simulink model "driver_model_b_upd (2)"  (R2023a)
settings: Solver=FixedStepDiscrete  StartTime=0  StopTime=700  FixedStep=0.0005  RelTol=1e-3  AbsTol=1e-6
InitFcn:
  | R2D = 180/pi;
undefined symbols (not defined in the file or in its folder): b_hat_Max, SrsLrn_BrkPedDownLim, SrsLrn_BrkPedUpLim, SrsLrn_EKF_Q1, SrsLrn_EKF_Q2, SrsLrn_ExitAccPedLim, SrsLrn_Lamda1, SrsLrn_Lamda2, SrsLrn_LongAccDownLim, SrsLrn_LongAccUpLim, SrsLrn_State1Cnt, SrsLrn_State2Cnt, SrsLrn_State5Cnt, SrsLrn_State6Cnt, SrsLrn_State7Cnt, SrsLrn_UpdBrkPedDown, SrsLrn_UpdBrkPedUp, tau_hat_Max
libraries: simulink x11, slpidlib x2, Solver_SF x1
(part 2 of 2)

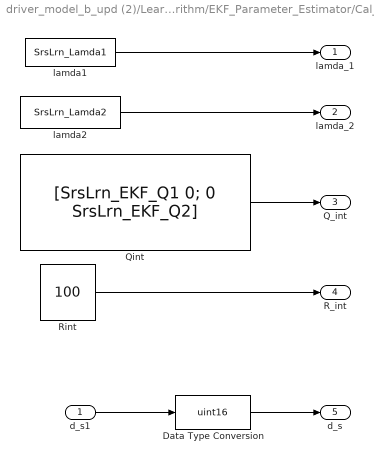
== system driver_model_b_upd (2)/LearningAlgorithm/EKF_Parameter_Estimator/Cal_para ==
  d_s1 : Inport
  Data Type Conversion : DataTypeConversion  OutDataTypeStr=uint16  SaturateOnIntegerOverflow=off  RndMeth=Floor
  Qint : Constant  Value=[SrsLrn_EKF_Q1 0; 0 SrsLrn_EKF_Q2]  OutDataTypeStr=fixdt(0,16,0.001,0)
  Rint : Constant  Value=100  OutDataTypeStr=fixdt(0,16,2)
  lamda1 : Constant  Value=SrsLrn_Lamda1
  lamda2 : Constant  Value=SrsLrn_Lamda2
  lamda_1 : Outport
  lamda_2 : Outport  Port=2
  Q_int : Outport  Port=3
  R_int : Outport  Port=4
  d_s : Outport  Port=5
  wires:
  lamda1/1 -> lamda_1/1
  Rint/1 -> R_int/1
  Qint/1 -> Q_int/1
  lamda2/1 -> lamda_2/1
  d_s1/1 -> Data Type Conversion/1
  Data Type Conversion/1 -> d_s/1

== stateflow chart driver_model_b_upd (2)/LearningAlgorithm/EKF_Parameter_Estimator/Initialize ==
  state Initialize
    en: y=0;
  state AfterInit
    en: y=1;
  (default) -> Initialize
  Initialize -> AfterInit
  data: y output

== stateflow chart driver_model_b_upd (2)/Chart ==
  state Accel_INIT_ON
    en:
    driver = uint8(0);
    srs =uint8(0);
    accel =uint8(0);
    accel_init = uint8(1);
  state SRS_ON
    en:
    driver = uint8(0);
    srs = uint8(1);
    SRSCnt=uint16(1);
    du:
    SRSCnt=SRSCnt+1;
    ex:
    SRSCnt=uint16(0);
  state Driver_ON
    en:
    driver = uint8(1);
    srs = uint8(0);
    DriverCnt=uint16(1);
    du:
    DriverCnt=DriverCnt+1;
    ex:
    DriverCnt=uint16(0);
  state Loop_State
    en:
    Loop=uint16(1);
    PreLoop = uint16(1);
  state INIT
    en:
    driver = uint8(0);
    srs =uint8(0);
    accel = uint8(0);
    accel_init = uint8(0);
    SRSCheck = uint16(0);
    DriverCnt=uint16(0);
  state Accel_ON
    en:
    driver = uint8(0);
    srs =uint8(0);
    accel = uint8(1);
    ACCCnt=uint16(1);
    du:
    ACCCnt=ACCCnt+1;
    ex:
    ACCCnt=uint16(0);
  state Loop_Update
    en:
    PreLoop = Loop;
    Loop=Loop+1;
    LoopCnt=uint16(1);
    du:
    LoopCnt=LoopCnt+1;
    ex:
    LoopCnt=uint16(0);
  state OFF
    en:
    driver = uint8(0);
    srs =uint8(0);
    accel = uint8(0);
  state Accel_OFF
    en:
    driver = uint8(0);
    srs =uint8(0);
    accel = uint8(0);
    ACCCnt=uint16(1);
    du:
    ACCCnt=ACCCnt+1;
    ex:
    ACCCnt=uint16(0);
  state Accel_INIT_OFF_L
    en:
    driver = uint8(0);
    srs =uint8(0);
    accel = uint8(0);
  state SRS_ON_L
    en:
    driver = uint8(0);
    srs = uint8(1);
    accel = uint8(0);
    SRSCnt=uint16(1);
    du:
    SRSCnt=SRSCnt+1;
    ex:
    SRSCnt=uint16(0);
  state Driver_ON_L
    en:
    driver = uint8(1);
    srs = uint8(0);
    accel = uint8(0);
    DriverCnt=uint16(1);
    du:
    DriverCnt=DriverCnt+1;
    ex:
    DriverCnt=uint16(0);
  state Accel_INIT_L
    en:
    driver = uint8(0);
    srs =uint8(0);
    accel = uint8(1);
    ACCCnt=uint16(1);
    du:
    ACCCnt=ACCCnt+1;
    ex:
    ACCCnt=uint16(0);
  state Accel_ON_L
    en:
    driver = uint8(0);
    srs =uint8(0);
    accel = uint8(1);
    ACCCnt=uint16(1);
    du:
    ACCCnt=ACCCnt+1;
    ex:
    ACCCnt=uint16(0);
  state Loop_Update_L
    en:
    PreLoop = Loop;
    Loop=Loop+1;
  state OFF_Driver_L
    en:
    driver = uint8(0);
    srs =uint8(0);
    accel = uint8(0);
  state Accel_OFF_L
    en:
    driver = uint8(0);
    srs =uint8(0);
    accel = uint8(0);
  (default) -> Loop_State
  SRS_ON -> Driver_ON : [(v_ego <1 && SRSCnt > 200) ||...
      |  (Pre_Vehicle_speed - v_ego >= 0 &&...
      |  SRSCnt > 200 ) ||...
      |  (d_des_driver > delta_d &&...
      |  SRSCnt > 200 )]
  INIT -> Accel_INIT_ON [order 2] : [Loop == 1 &&...
      |  D_des_SRS < delta_d &&...
      |  clock >=0]
  Accel_INIT_ON -> SRS_ON : [throttle_input == 0 &&...
      | Pre_Vehicle_speed - v_ego < 0  &&...
      |  D_des_SRS > delta_d ]
  Loop_State -> INIT
  Driver_ON -> OFF : [(d_des_driver <= delta_d  &&...
      |  clock < 100 &&...
      | DriverCnt > 50) ||...
      | clock >= 100*Loop]
  OFF -> Driver_ON [order 1] : [Pre_Vehicle_speed - v_ego < 3 &&...
      | d_des_driver > delta_d  &&...
      | clock <100 *Loop  ]
  Accel_ON -> INIT [order 2] : [clock >= 200*PreLoop]
  OFF -> Loop_Update [order 2] : [clock >=100*Loop]
  Accel_ON -> Accel_OFF [order 1] : [( v_ego - Pre_Vehicle_speed  > 3 &&...
      |  ACCCnt >100 ) ||...
      |  delta_d <= 15  ]
  Accel_OFF -> Accel_ON [order 1] : [D_des_SRS < delta_d &&...
      | clock >= 100 &&...
      | delta_d >=70]
  Loop_Update -> (junction 292)
  (junction 292) -> Accel_OFF
  Accel_OFF -> INIT [order 2] : [clock >= PreLoop*200]
  Accel_INIT_OFF_L -> (junction 288) [order 1] : [Pre_Vehicle_speed - v_ego < 0  &&...
      |  D_des_SRS > delta_d]
  (junction 288) -> SRS_ON_L
  Accel_INIT_OFF_L -> Accel_INIT_L [order 2] : [D_des_SRS < delta_d &&...
      | delta_d > 80]
  Accel_INIT_L -> Accel_INIT_OFF_L : [ACCCnt == 200 ||...
      |  delta_d < 10 ||...
      | D_des_SRS +20 >= delta_d ||...
      | (v_ego >=18 && ACCCnt == 200)]
  SRS_ON_L -> Driver_ON_L : [(v_ego <1 && SRSCnt >100) ||...
      |  (Pre_Vehicle_speed - v_ego <= 0 &&...
      | d_des_driver >= delta_d &&...
      |  SRSCnt > 100) ||...
      |  (d_des_driver > delta_d &&...
      |  SRSCnt > 100 )]
  INIT -> Accel_INIT_L [order 1] : [Loop == (PreLoop+1)&&...
      |  D_des_SRS <= delta_d &&...
      | clock >=100*Loop]
  (junction 211) -> SRS_ON_L
  Driver_ON_L -> OFF_Driver_L : [(d_des_driver <= delta_d &&...
      | DriverCnt > 50 &&...
      | Pre_Vehicle_speed - v_ego >= 0 &&...
      | clock < (100+PreLoop*200))||...
      | clock >= (100+PreLoop*200) ||...
      | d_des_driver <= delta_d ]
  OFF_Driver_L -> Driver_ON_L [order 2] : [(clock < (100+PreLoop*200) &&...
      |  Pre_Vehicle_speed - v_ego < 0 &&...
      |  d_des_driver > delta_d )]
  INIT -> (junction 211) [order 3] : [Loop==(PreLoop+1) &&...
      | Pre_Vehicle_speed - v_ego < 0  &&...
      |  D_des_SRS > delta_d &&...
      |  clock >=100*Loop + 15]
  Accel_ON_L -> INIT [order 2] : [clock >=PreLoop*200]
  OFF_Driver_L -> Loop_Update_L [order 1] : [clock >=200*PreLoop+100]
  Accel_ON_L -> Accel_OFF_L [order 1] : [(v_ego - Pre_Vehicle_speed  > 3 &&...
      | clock < PreLoop*200 &&...
      |  ACCCnt >100 ) ||...
      |  (clock < PreLoop*200 &&...
      | delta_d < 15) ]
  Accel_OFF_L -> Accel_ON_L [order 1] : [D_des_SRS < delta_d &&...
      | clock < PreLoop*200 &&...
      | delta_d >=70]
  Loop_Update_L -> (junction 290)
  (junction 290) -> Accel_OFF_L
  Accel_OFF_L -> INIT [order 2] : [clock >=PreLoop*200]
  data: d_des_driver input; srs output; driver output; accel output; v_ego input; D_des_SRS input; delta_d input; Pre_Vehicle_speed input; DriverCnt local; throttle_input input; SRSCnt local; SRSCheck local; clock input; ACCCnt local; accelCheck local; LoopCnt local; accel_init local; BrakeCnt local; Loop output; DoCnt local; STCnt local; PreLoop local

== stateflow chart driver_model_b_upd (2)/LearningAlgorithm/EKF_Parameter_Estimator/Initialize1 ==
  state Initialize
    en: y=0;
  state AfterInit
    en: y=1;
  (default) -> Initialize
  Initialize -> AfterInit
  data: y output

== stateflow chart driver_model_b_upd (2)/LearningAlgorithm/SRS_Learning_State ==
  state SRSBrkLrnEna
    en:
    SrsLrn_state=uint8(5);
  state Init
    en:
    SrsLrn_state=uint8(0);
  state SRSBrk_ConsAcc
    en:
    BCCnt = uint16(1);
    du:
    BCCnt = BCCnt + 1;
    ex:
    BCCnt = uint16(0);
    state BrkTau_Update
      en:
      SrsLrn_state=uint8(3);
    state Brkb_Update
      en:
      SrsLrn_state=uint8(4);
    (default) -> (junction 94)
    (junction 94) -> BrkTau_Update [order 1] : [RelSpdDivVego < 0.01]
    (junction 94) -> Brkb_Update [order 2] : [RelSpdDivVego > 0.01]
  note: % Brake Pedal 변화 3%미만, Acc 변화 50% 미만
      | [DBCnt > SrsLrn_State2Cnt &&...
      | StrkDpthPcVal < SrsLrn_BrkPedUpLim*BrkStrk &&...
      | StrkDpthPcVal > SrsLrn_BrkPedDownLim*BrkStrk]
      |
      | % 종방향 가속도 조건은 필요시 추가 (종방향 가속도 음수 상황)
      | % LongAccFil > SrsLrn_LongAccDownLim*AccVal &&...
      | % LongAccFil < SrsLrn_LongAccUpLim*AccVal]
  state SRSDriverBrk
    en:
    SrsLrn_state=uint8(2);
    DBCnt = uint16(1);
    BrkStrk = StrkDpthPcVal;
    % AccVal = LongAccFil;
    du:
    DBCnt = DBCnt + 1;
    ex:
    DBCnt = uint16(0);
  state SRSCarfollow
    en:
    SrsLrn_state=uint8(1);
    CfCnt = uint16(1);
    du:
    CfCnt = CfCnt + 1;
    ex:
    CfCnt = uint16(0);
  state SRSDriverAcc
    en:
    SrsLrn_state=uint8(6);
    DBCnt_Acc= uint16(1);
    AccVal = LongAccFil;
    du:
    DBCnt_Acc = DBCnt_Acc + 1;
    ex:
    DBCnt_Acc = uint16(0);
  state SRSAcc_AccUp
    en:
    SrsLrn_state=uint8(7);
    BCCnt_Acc = uint16(1);
    du:
    BCCnt_Acc = BCCnt_Acc + 1;
    ex:
    BCCnt_Acc = uint16(0);
  state SRSAccLrnEna
    en:
    AccCnt = uint16(1);
    AccPed = AccPedDepVal;
    du:
    AccCnt = AccCnt + 1;
    ex:
    AccCnt = uint16(0);
    state AccTau_Update
      en:
      SrsLrn_state=uint8(8);
    state Accb_Update
      en:
      SrsLrn_state=uint8(9);
    (default) -> (junction 100)
    (junction 100) -> AccTau_Update [order 1] : [RelSpdDivVego < 0.05]
    (junction 100) -> Accb_Update [order 2] : [RelSpdDivVego > 0.05]
  (default) -> Init
  SRSBrkLrnEna -> Init : [SmartRegenRdrCstActSta ==0 ||...
      |  AccPedDepVal > 2 ||...
      | ObjDstVal > 100 ||...
      | sEstSpdFilt < 0.5 ||...
      | StrkDpthPcVal > 0.5 ||...
      | ObjRelSpdVal > 0.1]
  SRSBrk_ConsAcc -> SRSBrkLrnEna [order 1] : [StrkDpthPcVal == 0]
  SRSBrk_ConsAcc -> Init [order 2] : [SmartRegenRdrCstActSta ==0 ||...
      |  AccPedDepVal > 2 ||...
      | ObjDstVal > 100 ||...
      | sEstSpdFilt < 0.5 ||...
      | ObjRelSpdVal > 0.1 ||...
      | StrkDpthPcVal > 1.5*BrkStrk ||...
      | StrkDpthPcVal < 0.5*BrkStrk]
      | % 종방향 가속도 조건은 필요시 추가 (종방향 가속도 음수 상황)
      | % LongAccFil < SrsLrn_LongAccDownLim*AccVal ||...
      | % LongAccFil > SrsLrn_LongAccUpLim*AccVal
  SRSDriverBrk -> SRSBrk_ConsAcc [order 2] : % Brake Pedal 변화 3%미만, Acc 변화 50% 미만
      | [DBCnt > SrsLrn_State2Cnt &&...
      | StrkDpthPcVal < 1.5*BrkStrk &&...
      | StrkDpthPcVal > 0.2*BrkStrk]
      |
      | % 종방향 가속도 조건은 필요시 추가 (종방향 가속도 음수 상황)
      | % LongAccFil > SrsLrn_LongAccDownLim*AccVal &&...
      | % LongAccFil < SrsLrn_LongAccUpLim*AccVal]
  SRSDriverBrk -> Init [order 1] : [SmartRegenRdrCstActSta ==0 ||...
      |  AccPedDepVal > 2 ||...
      | ObjDstVal > 100 ||...
      | sEstSpdFilt < 0.5 ||...
      | ObjRelSpdVal > 0.1 ]
  SRSDriverBrk -> (junction 43) [order 4] : [StrkDpthPcVal > 1.5*BrkStrk ||...
      | StrkDpthPcVal < 0.2*BrkStrk]
  (junction 43) -> SRSDriverBrk
  SRSDriverBrk -> (junction 26) [order 3]
  (junction 26) -> SRSCarfollow : [SmartRegenRdrCstActSta == 1 &&...
      | MotTqCmdRearVal <0 &&...
      | sEstSpdFilt > 1 &&...
      | ObjDstVal < 60 &&...
      | ObjDstVal < SrsCfc_dTgt &&...
      | ObjRelSpdVal < 0 &&...
      | StrkDpthPcVal < 0.5 &&...
      | AccPedDepVal < 0.5]
  (junction 9) -> SRSDriverBrk : [CfCnt >SrsLrn_State1Cnt &&...
      | StrkDpthPcVal > 5]
  Init -> SRSCarfollow : [SmartRegenRdrCstActSta ==1 &&...
      | MotTqCmdRearVal <0 &&...
      | sEstSpdFilt > 1 &&...
      | ObjDstVal < 60 &&...
      | ObjDstVal > 0.5 &&...
      | ObjDstVal < SrsCfc_dTgt &&...
      | ObjRelSpdVal < -0.01 &&...
      | StrkDpthPcVal < 0.5 &&...
      | AccPedDepVal < 0.5]
  SRSCarfollow -> (junction 9) [order 1]
  SRSCarfollow -> Init [order 3] : [SmartRegenRdrCstActSta ==0 ||...
      |  AccPedDepVal > 2 ||...
      | ObjDstVal > 100 ||...
      | sEstSpdFilt < 0.5 ||...
      | ObjRelSpdVal > 0.1]
  SRSCarfollow -> (junction 75) [order 2]
  (junction 75) -> SRSDriverAcc : [CfCnt> SrsLrn_State1Cnt &&...
      | AccPedDepVal > 1]
  (junction 69) -> SRSCarfollow : [SmartRegenRdrCstActSta == 1 &&...
      | MotTqCmdRearVal < 0 &&...
      | sEstSpdFilt > 1 &&...
      | ObjDstVal < 60 &&...
      | ObjDstVal > 0 &&...
      | ObjDstVal < SrsCfc_dTgt &&...
      | ObjRelSpdVal < 0 &&...
      | StrkDpthPcVal < 5 &&...
      | AccPedDepVal < 0.05]
  SRSDriverAcc -> (junction 69) [order 1]
  SRSDriverAcc -> Init [order 3] : [SmartRegenRdrCstActSta ==0 ||...
      | StrkDpthPcVal > 2 ||...
      | ObjDstVal > 100 ||...
      | sEstSpdFilt < 0.5 ||...
      | ObjRelSpdVal > 0 ||...
      | ObjRelSpdVal == 0 ||...
      | AccPedDepVal == 0]
  SRSDriverAcc -> SRSAcc_AccUp [order 2] : [ %State5에 머무르는 시간
      | %AccPedDepVal > 5 의 경우 실차 데이터 기준으로 5
      | %CarSim Accel 시나리오의 경우 AccPedDepVal > 2.5로 수정해야 학습 진행
      | DBCnt_Acc > SrsLrn_State5Cnt &&...
      | AccPedDepVal > 5 &&...
      | AccPedDepVal > AccPedDepVal_z]
  SRSAcc_AccUp -> Init [order 1] : [SmartRegenRdrCstActSta == 0 ||...
      | StrkDpthPcVal > 2 ||...
      | ObjDstVal > 100 ||...
      | sEstSpdFilt < 0.5 ||...
      | ObjRelSpdVal > 0 ||...
      | ObjRelSpdVal == 0 ||...
      | AccPedDepVal == 0]
  SRSAcc_AccUp -> SRSAccLrnEna [order 2] : [BCCnt_Acc > SrsLrn_State6Cnt &&...
      | AccPedDepVal < AccPedDepVal_z]
  SRSAccLrnEna -> Init : [SmartRegenRdrCstActSta ==0  ||...
      | StrkDpthPcVal > 2 ||...
      | ObjDstVal > 100 ||...
      | sEstSpdFilt < 0.5 ||...
      | AccPedDepVal == 0 ||...
      | ObjRelSpdVal > 0 ||...
      | ObjRelSpdVal == 0 ||...
      | AccCnt > SrsLrn_State7Cnt ||...
      | AccPedDepVal < SrsLrn_ExitAccPedLim*AccPed]
  data: SmartRegenRdrCstActSta input; ObjDstVal input; MotTqCmdRearVal input; SrsCfc_dTgt input; sEstSpdFilt input; ObjRelSpdVal input; RelSpdDivVego input; AccPedDepVal input; StrkDpthPcVal input; SrsLrn_state output uint8; CfCnt local uint16; DBCnt local uint16; BCCnt local uint16; LongAccFil input; AccVal local; BrkStrk local; SrsLrn_State1Cnt parameter uint16; SrsLrn_UpdBrkPedUp parameter fixdt(1,16,9); SrsLrn_UpdBrkPedDown parameter fixdt(1,16,9); SrsLrn_State2Cnt parameter double; SrsLrn_BrkPedUpLim parameter fixdt(1,16,9); SrsLrn_BrkPedDownLim parameter fixdt(1,16,9); SrsLrn_LongAccDownLim parameter fixdt(1,16,9); SrsLrn_LongAccUpLim parameter fixdt(1,16,9); SrsLrn_State5Cnt parameter uint16; SrsLrn_State6Cnt parameter uint16; SrsLrn_State7Cnt parameter uint16; SrsLrn_ExitAccPedLim parameter fixdt(1,16,9); AccPedDepVal_z input; BCCnt_Acc local uint16; DBCnt_Acc local uint16; AccPed local; AccCnt local uint16

== stateflow chart driver_model_b_upd (2)/LearningAlgorithm/EKF_Parameter_Estimator/Initialize2 ==
  state Initialize
    en: y=0;
  state AfterInit
    en: y=1;
  (default) -> Initialize
  Initialize -> AfterInit
  data: y output
